simulink model "PitchControl"  (R2022b)
settings: Solver=VariableStepAuto  StartTime=0.0  StopTime=40  RelTol=1e-3
undefined symbols (not defined in the file or in its folder): den_q_sp, den_theta, num_q_sp, num_theta
settings Model: Creator=^-^  LastModifiedBy=^-^

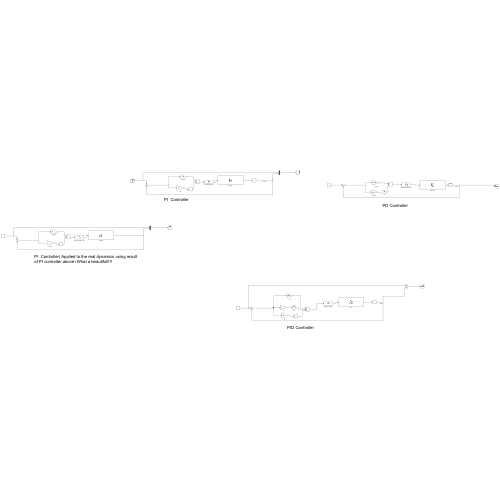
[thumbnail: Simulink's stored preview of the top-level diagram]
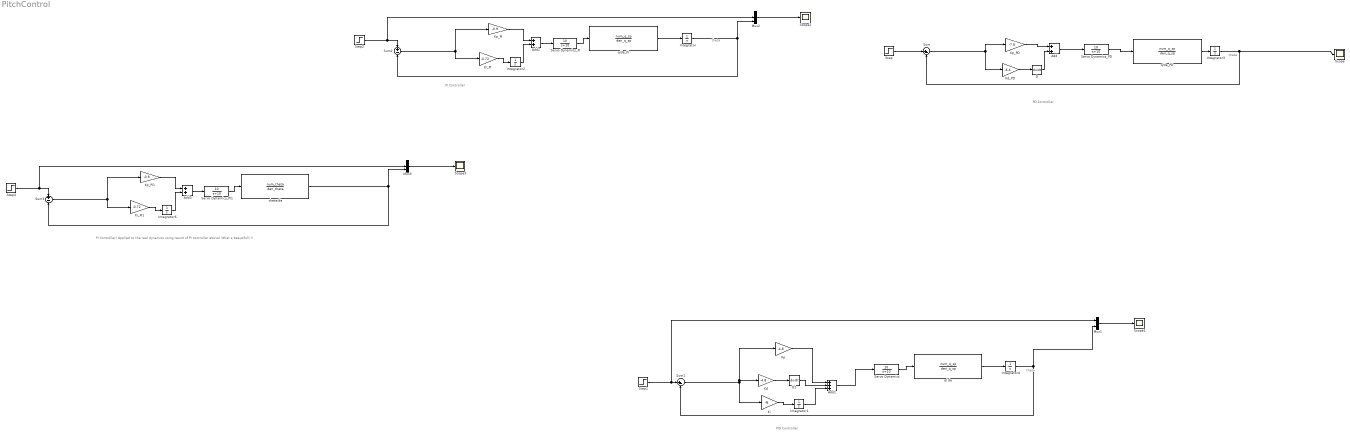
== system PitchControl ==
  note: theta
  note: theta
  note: theta
  note: PID Controller
  note: PD Controller
  note: PI Controller
  note: PI Controller( Applied to the real dynamics using result of PI controller above) What a beautiful!!!!
  Add : Sum
  Add1 : Sum  Inputs=+++
  Add2 : Sum
  Add3 : Sum
  D : Derivative
  D1 : Derivative
  Integrator{,1..4,6} (6 alike) : Integrator
  Kd : Gain  Gain=-4.8
  Kd_PD : Gain  Gain=-6.4
  Ki : Gain  Gain=-6
  Ki_PI : Gain  Gain=-0.72
  Ki_PI1 : Gain  Gain=-0.72
  Kp : Gain  Gain=-4.8
  Kp_PD : Gain  Gain=-7.8
  Kp_PI : Gain  Gain=-0.9
  Kp_PI1 : Gain  Gain=-0.9
  Mux1 : Mux  Inputs=2
  Mux2 : Mux  Inputs=3
  Mux3 : Mux  Inputs=3
  Scope{,1..3} (4 alike) : Scope
  Servo Dynamics : TransferFcn  Numerator=10  Denominator=[1 10]
  Servo Dynamics_PD : TransferFcn  Numerator=10  Denominator=[1 10]
  Servo Dynamics_PI : TransferFcn  Numerator=10  Denominator=[1 10]
  Servo Dynamics_PI1 : TransferFcn  Numerator=10  Denominator=[1 10]
  Step{,1..3} (4 alike) : Step  SampleTime=0
  Sum : Sum  Inputs=|+-
  Sum1 : Sum  Inputs=|+-
  Sum2 : Sum  Inputs=+-
  Sum3 : Sum  Inputs=+-
  q/ de : TransferFcn  Numerator=num_q_sp  Denominator=den_q_sp
  q/de_PD : TransferFcn  Numerator=num_q_sp  Denominator=den_q_sp
  q/de_PI : TransferFcn  Numerator=num_q_sp  Denominator=den_q_sp
  theta/de : TransferFcn  Numerator=num_theta  Denominator=den_theta
  wires:
  D/1 -> Add/2
  Kp_PD/1 -> Add/1
  Step/1 -> Sum/1
  Sum/1 -> Kp_PD/1, Kd_PD/1
  Kd_PD/1 -> D/1
  Integrator2/1 -> Add2/2
  Step2/1 -> Mux2/2, Sum2/1
  Integrator/1 -> Mux2/3, Sum2/2
  Sum2/1 -> Kp_PI/1, Ki_PI/1
  Mux2/1 -> Scope2/1
  Kp_PI/1 -> Add2/1
  Ki_PI/1 -> Integrator2/1
  Sum1/1 -> Kd/1, Kp/1, Ki/1
  Kd/1 -> D1/1
  Integrator4/1 -> Sum1/2, Mux1/2
  Mux1/1 -> Scope1/1
  D1/1 -> Add1/2
  Integrator1/1 -> Add1/3
  Kp/1 -> Add1/1
  Ki/1 -> Integrator1/1
  Step1/1 -> Mux1/1, Sum1/1
  Integrator3/1 -> Scope/1, Sum/2
  Add2/1 -> Servo Dynamics_PI/1
  Servo Dynamics_PI/1 -> q/de_PI/1
  Servo Dynamics_PD/1 -> q/de_PD/1
  Add/1 -> Servo Dynamics_PD/1
  Add1/1 -> Servo Dynamics/1
  Servo Dynamics/1 -> q/ de/1
  q/de_PI/1 -> Integrator/1
  q/de_PD/1 -> Integrator3/1
  q/ de/1 -> Integrator4/1
  Step3/1 -> Mux3/2, Sum3/1
  Kp_PI1/1 -> Add3/1
  Servo Dynamics_PI1/1 -> theta/de/1
  Add3/1 -> Servo Dynamics_PI1/1
  Ki_PI1/1 -> Integrator6/1
  Sum3/1 -> Kp_PI1/1, Ki_PI1/1
  Integrator6/1 -> Add3/2
  theta/de/1 -> Mux3/3, Sum3/2
  Mux3/1 -> Scope3/1
